simulink model "test_mtimes"  (R2020b)
settings: Solver=FixedStepDiscrete  StartTime=0.0  StopTime=10.0  FixedStep=0.100000  RelTol=1e-3
model workspace (MAT data in the model file):
  already_pp = 1
settings Model: Creator=fconzelm  LastModifiedBy=hbourbou
settings DataIOCC: ReturnWorkspaceOutputs=off
settings DebuggingCC: AlgebraicLoopMsg=error  ArtificialAlgebraicLoopMsg=error  SaveWithDisabledLinksMsg=none  SingleTaskRateTransMsg=error  ArithmeticOperatorsInVariantConditions=warning
settings SFSimCC: SimUseLocalCustomCode=off  CustomCodeUndefinedFunction=UseInterfaceOnly
settings RTWCC: RTWUseLocalCustomCode=off

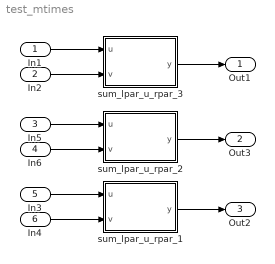
== system test_mtimes ==
  In1 : Inport  PortDimensions=[1 1]
  In2 : Inport  Port=2  PortDimensions=[3 2]
  In5 : Inport  Port=3  PortDimensions=[1 3]
  In6 : Inport  Port=4  PortDimensions=[3 2]
  In3 : Inport  Port=5  PortDimensions=[3 2]
  In4 : Inport  Port=6  PortDimensions=[2 3]
  sum_lpar_u_rpar_1 : MATLAB Function  TreatAsAtomicUnit=on
  sum_lpar_u_rpar_2 : MATLAB Function  TreatAsAtomicUnit=on
  sum_lpar_u_rpar_3 : MATLAB Function  TreatAsAtomicUnit=on
  Out1 : Outport  VectorParamsAs1DForOutWhenUnconnected=off
  Out3 : Outport  Port=2  VectorParamsAs1DForOutWhenUnconnected=off
  Out2 : Outport  Port=3  VectorParamsAs1DForOutWhenUnconnected=off
  wires:
  In1/1 -> sum_lpar_u_rpar_3/1(u)
  sum_lpar_u_rpar_3/1(y) -> Out1/1
  In2/1 -> sum_lpar_u_rpar_3/2(v)
  In6/1 -> sum_lpar_u_rpar_2/2(v)
  In5/1 -> sum_lpar_u_rpar_2/1(u)
  sum_lpar_u_rpar_2/1(y) -> Out3/1
  In4/1 -> sum_lpar_u_rpar_1/2(v)
  In3/1 -> sum_lpar_u_rpar_1/1(u)
  sum_lpar_u_rpar_1/1(y) -> Out2/1

== matlab function test_mtimes/sum_lpar_u_rpar_2 ==
  data: u input; y output; v input
function y = mtimes1(u, v)

y = mtimes(u, v);

== matlab function test_mtimes/sum_lpar_u_rpar_3 ==
  data: u input; y output; v input
function y = mtimes1(u, v)

y = mtimes(u, v);

== matlab function test_mtimes/sum_lpar_u_rpar_1 ==
  data: u input; y output; v input
function y = mtimes1(u, v)

y = u * v;
